simulink model "Modelo_con_no_linealidades_filtro_sensor"  (R2020a)
settings: Solver=ode15s  StartTime=0.0  StopTime=10  FixedStep=0.001  MaxStep=0.0001  RelTol=1e-3
undefined symbols (not defined in the file): A, Amp, B, ba, Cc, D, den_anti, den_des, den_mems, den_piezo, f0, fs, g, I_max, K_motor_virtual, ksi, ksia, L, num_anti, num_des, num_mems, num_piezo, R, R_control, sens_mems, sens_piezo, v0, Vcc, x0, ZOH
libraries: simulink x2, dsparch4 x2, simulink_extras x2, dspstat3 x1
settings Model: Creator=Noxi-PC  LastModifiedBy=Noxi-PC

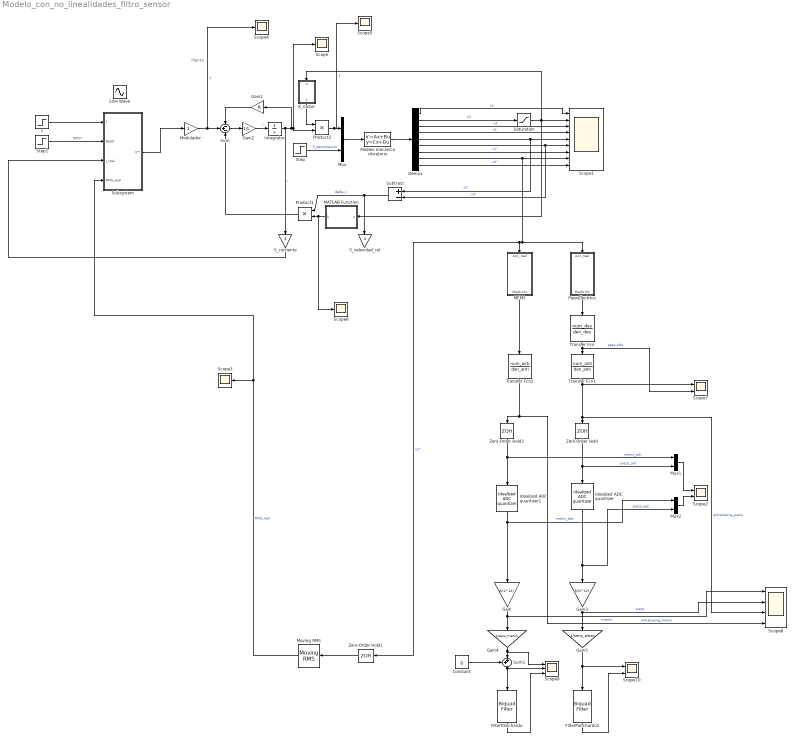
== system Modelo_con_no_linealidades_filtro_sensor ==
  note: Planta
  " PiezoElectrico" : Subsystem
  Constant : Constant  Value=g
  Demux : Demux  Outputs=9
  FilterPanchardo : dsparch4/Biquad Filter  Tag=BlockMethodSubSystem  FilterSource=Dialog parameters  CoeffSource=Specify via dialog  FilterObject=BQF  IIRFiltStruct=Direct form II  BiQuadCoeffs=[1 0 -1 1 -1.99807727905716614 0.999282800663373716;1 0 -1 1 -1.9986275895624166 0.999418888027123309;1 0 -1 1 -1.9966899219313865 0.997885027756237442;1 0 -1 1 -1.99747521879656054 0.998272398940524885;1 0 -1 1 -1.99541616433952562 0.996591907571157343;1 0 -1 1 -1.9963625045137694 0.997171843682499337;1 0 -1 1 -1.99431507711195533 0.995463604360754095;1 0 -1 1 -1.99532069965140524 0.996148326323776701;1 0 -1 1 -1.9934341214911746 0.99454907245261337;1 0 -1 1 -1.99438289828679416 0.995234669646854031;1 0 -1 1 -1.99280645736345186 0.993883243383688608;1 0 -1 1 -1.99358390398571439 0.994465232331816384;1 0 -1 1 -1.9924496211917011 0.993485563750365785;1 0 -1 1 -1.99295923065970682 0.993874854162103194;1 0 -1 1 -1.99236572677773305 0.993360052380677261;1 0 -1 1 -1.99254312887680385 0.993496835183648508]  ScaleValues=[0.00331146928203063717;0.00331146928203063717;0.00330936361502479461;0.00330936361502479461;0.00330738378960852624;0.00330738378960852624;0.00330560502842379075;0.00330560502842379075;0.00330409457240921122;0.00330409457240921122;0.00330290926614940734;0.00330290926614940734;0.00330209355456580114;0.00330209355456580114;0.00330167794092392887;0.00330167794092392887;1]  IC=0  ICnum=0  ICden=0  a0Flag=Warning  optimizeScaleValues=on  ScaleValueMode=Specify via input port (g)  InputProcessing=Columns as channels (frame based)  roundingMode=Floor  overflowMode=off  scaleValueFracLength=14  denProdOutputFracLength=30  denAccumFracLength=30  secondMemoryFracLength=15
  FilterPanchardo1 : dsparch4/Biquad Filter  Tag=BlockMethodSubSystem  FilterSource=Dialog parameters  CoeffSource=Specify via dialog  FilterObject=BQF  IIRFiltStruct=Direct form II  BiQuadCoeffs=[1 0 -1 1 -1.99807727905716614 0.999282800663373716;1 0 -1 1 -1.9986275895624166 0.999418888027123309;1 0 -1 1 -1.9966899219313865 0.997885027756237442;1 0 -1 1 -1.99747521879656054 0.998272398940524885;1 0 -1 1 -1.99541616433952562 0.996591907571157343;1 0 -1 1 -1.9963625045137694 0.997171843682499337;1 0 -1 1 -1.99431507711195533 0.995463604360754095;1 0 -1 1 -1.99532069965140524 0.996148326323776701;1 0 -1 1 -1.9934341214911746 0.99454907245261337;1 0 -1 1 -1.99438289828679416 0.995234669646854031;1 0 -1 1 -1.99280645736345186 0.993883243383688608;1 0 -1 1 -1.99358390398571439 0.994465232331816384;1 0 -1 1 -1.9924496211917011 0.993485563750365785;1 0 -1 1 -1.99295923065970682 0.993874854162103194;1 0 -1 1 -1.99236572677773305 0.993360052380677261;1 0 -1 1 -1.99254312887680385 0.993496835183648508]  ScaleValues=[0.00331146928203063717;0.00331146928203063717;0.00330936361502479461;0.00330936361502479461;0.00330738378960852624;0.00330738378960852624;0.00330560502842379075;0.00330560502842379075;0.00330409457240921122;0.00330409457240921122;0.00330290926614940734;0.00330290926614940734;0.00330209355456580114;0.00330209355456580114;0.00330167794092392887;0.00330167794092392887;1]  IC=0  ICnum=0  ICden=0  a0Flag=Warning  optimizeScaleValues=on  ScaleValueMode=Specify via input port (g)  InputProcessing=Columns as channels (frame based)  roundingMode=Floor  overflowMode=off  scaleValueFracLength=14  denProdOutputFracLength=30  denAccumFracLength=30  secondMemoryFracLength=15
  Gain : Gain  Gain=5/(2^12)
  Gain1 : Gain  Gain=R
  Gain2 : Gain  Gain=1/L
  Gain3 : Gain  Gain=5/(2^12)
  Gain4 : Gain  Gain=1/sens_mems
  Gain5 : Gain  Gain=1/sens_piezo
  Idealized ADC quantizer : simulink_extras/Additional Discrete/Idealized ADC quantizer  NumberOfConverterBits=12  Vmin=-2.5  Vmax=2.5  OutputDataType=int16  OutputNegativeValues=on
  Idealized ADC quantizer1 : simulink_extras/Additional Discrete/Idealized ADC quantizer  NumberOfConverterBits=12  Vmin=0  Vmax=3.3  OutputDataType=int16  OutputNegativeValues=on
  Integrator : Integrator
  K_motor : MATLAB Function  TreatAsAtomicUnit=on
  MATLAB Function : MATLAB Function  TreatAsAtomicUnit=on
  MEMS : Subsystem
  Modelo mecánico vibratorio : StateSpace  A=A  B=B  C=Cc  D=D  InitialCondition=[x0,v0]
  Modulador : Gain
  Moving RMS : dspstat3/Moving RMS  Method=Sliding window  ForgettingFactorPort=off  SpecifyWindowLength=on  WindowLength=Ventana  ForgettingFactor=0.99  SimulateUsing=Code generation
      settings: SourceProductBaseCode=DS
  Mux : Mux  Inputs=2
  Mux1 : Mux  Inputs=2
  Mux2 : Mux  Inputs=2
  Product1 : Product
  Product2 : Product
  S_corriente : Gain
  S_velocidad_rel : Gain
  Saturation : Saturate  UpperLimit=12.7e-3  LowerLimit=-12.7e-3
  Scope{,3..6} (5 alike) : Scope
  Scope1 : Scope  NumInputPorts=9
  Scope10 : Scope  NumInputPorts=2
  Scope2 : Scope  NumInputPorts=2
  Scope7 : Scope  NumInputPorts=2
  Scope8 : Scope  NumInputPorts=4
  Scope9 : Scope  NumInputPorts=3
  Sine Wave : Sin  Amplitude=5  Frequency=2*pi*f0  SampleTime=0
  Step : Step  Time=3  After=0  SampleTime=0
  Step1 : Step  After=Amp/sqrt(2)  SampleTime=0
  Subsystem : Subsystem
  Subtract : Sum  Inputs=+-
  Sum : Sum  Inputs=-+-
  Sum1 : Sum  Inputs=++|
  Transfer Fcn : TransferFcn  Numerator=num_des  Denominator=den_des
  Transfer Fcn1 : TransferFcn  Numerator=num_anti  Denominator=den_anti
  Transfer Fcn2 : TransferFcn  Numerator=num_anti  Denominator=den_anti
  Zero-Order Hold : ZeroOrderHold  SampleTime=1/fs
  Zero-Order Hold1 : ZeroOrderHold  SampleTime=ZOH
  Zero-Order Hold2 : ZeroOrderHold  SampleTime=1/fs
  f : Step  Time=0  After=f0  SampleTime=0
  wires:
  Modelo mecánico vibratorio/1 -> Demux/1
  Demux/1 -> Scope1/1  "x1"
  Demux/2 -> Saturation/1  "x2"
  Demux/3 -> Scope1/3  "x3"
  Demux/4 -> Scope1/4  "x1'"
  Demux/5 -> Scope1/5, Subtract/1  "x2'"
  Demux/6 -> Scope1/6, Subtract/2  "x3'"
  Demux/7 -> Scope1/7  "x1''"
  Demux/8 -> " PiezoElectrico"/1(Acc_real), Zero-Order Hold1/1, MEMS/1(Acc_real), Scope1/8  "x2''"
  Demux/9 -> Scope1/9  "x3''"
  Mux/1 -> Modelo mecánico vibratorio/1
  Sum/1 -> Gain2/1
  Integrator/1 -> S_corriente/1, Product2/2, Scope/1, Gain1/1  "i"
  Gain1/1 -> Sum/1
  Gain2/1 -> Integrator/1  "i'"
  Step/1 -> Mux/2  "F_perturbación"
  Product1/1 -> Sum/3
  Subtract/1 -> Product1/1, S_velocidad_rel/1  "delta_v"
  Modulador/1 -> Scope4/1, Sum/2  "V"
  Moving RMS/1 -> Subsystem/4(RMS_real), Scope3/1  "RMS_real"
  Saturation/1 -> K_motor/1(u), MATLAB Function/1(u), Scope1/2
  Product2/1 -> Scope5/1, Mux/1  "F"
  K_motor/1(k) -> Product2/1
  MATLAB Function/1(k) -> Scope6/1, Product1/2
  f/1 -> Subsystem/1(f)
  Step1/1 -> Subsystem/2(RMS*)  "RMS*"
  S_corriente/1 -> Subsystem/3(i_real)
  Subsystem/1(V*') -> Modulador/1
  " PiezoElectrico"/1(Medición) -> Transfer Fcn/1
  Transfer Fcn/1 -> Scope7/2, Transfer Fcn1/1  "pasa-alto"
  Transfer Fcn1/1 -> Scope8/3, Zero-Order Hold/1, Scope7/1  "antialiasing_piezo"
  Zero-Order Hold/1 -> Mux1/2, Idealized ADC quantizer/1  "piezo_zoh"
  MEMS/1(Medición) -> Transfer Fcn2/1
  Transfer Fcn2/1 -> Scope8/4, Zero-Order Hold2/1  "antialiasing_mems"
  Zero-Order Hold2/1 -> Mux1/1, Idealized ADC quantizer1/1  "mems_zoh"
  Mux1/1 -> Scope2/1
  Idealized ADC quantizer/1 -> Mux2/2, Gain3/1  "piezo_adc"
  Idealized ADC quantizer1/1 -> Gain/1, Mux2/1  "mems_adc"
  Mux2/1 -> Scope2/2
  Gain/1 -> Scope8/1, Gain4/1  "mems"
  Gain3/1 -> Scope8/2, Gain5/1  "piezo"
  Sum1/1 -> Scope9/2, FilterPanchardo/1
  Gain4/1 -> Scope9/1, Sum1/2
  Constant/1 -> Sum1/1
  Gain5/1 -> FilterPanchardo1/1, Scope10/1
  FilterPanchardo1/1 -> Scope10/2
  FilterPanchardo/1 -> Scope9/3
  Zero-Order Hold1/1 -> Moving RMS/1

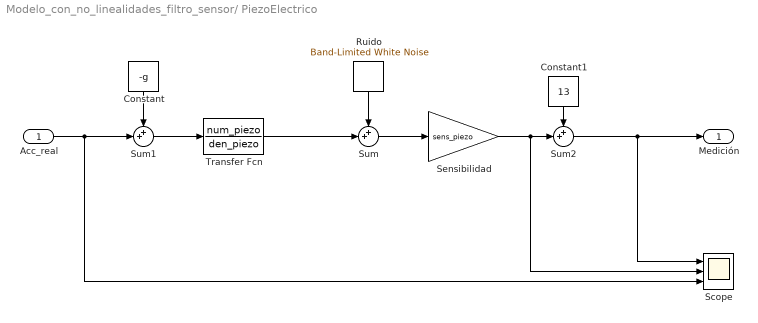
== system Modelo_con_no_linealidades_filtro_sensor/ PiezoElectrico ==
  Acc_real : Inport
  Constant : Constant  Value=-g
  Constant1 : Constant  Value=13
  Ruido : simulink/Sources/Band-Limited White Noise  Cov=NoisePower_piezo  Ts=1/fs  seed=[23341]
  Scope : Scope  NumInputPorts=3
  Sensibilidad : Gain  Gain=sens_piezo
  Sum : Sum  Inputs=++|
  Sum1 : Sum  Inputs=++|
  Sum2 : Sum  Inputs=++|
  Transfer Fcn : TransferFcn  Numerator=num_piezo  Denominator=den_piezo
  Medición : Outport
  wires:
  Transfer Fcn/1 -> Sum/2
  Ruido/1 -> Sum/1
  Constant/1 -> Sum1/1
  Sum1/1 -> Transfer Fcn/1
  Acc_real/1 -> Scope/3, Sum1/2
  Sum/1 -> Sensibilidad/1
  Constant1/1 -> Sum2/1
  Sensibilidad/1 -> Scope/2, Sum2/2
  Sum2/1 -> Medición/1, Scope/1

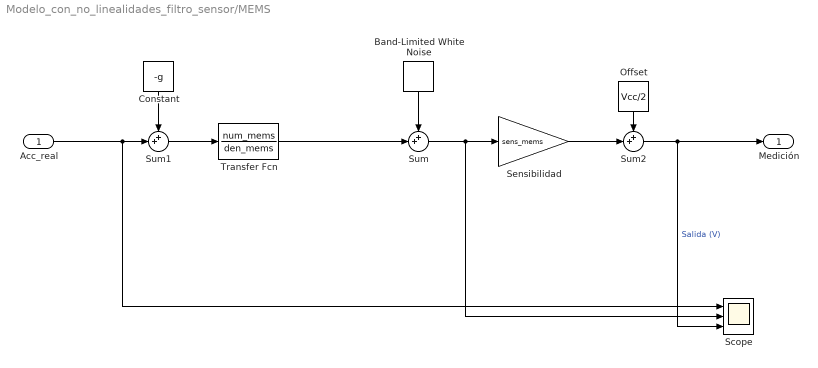
== system Modelo_con_no_linealidades_filtro_sensor/MEMS ==
  Acc_real : Inport
  Band-Limited White Noise : simulink/Sources/Band-Limited White Noise  Cov=NoisePower_mems  Ts=1/fs  seed=[23341]
  Constant : Constant  Value=-g
  Offset : Constant  Value=Vcc/2
  Scope : Scope  NumInputPorts=3
  Sensibilidad : Gain  Gain=sens_mems
  Sum : Sum  Inputs=++|
  Sum1 : Sum  Inputs=++|
  Sum2 : Sum  Inputs=++|
  Transfer Fcn : TransferFcn  Numerator=num_mems  Denominator=den_mems
  Medición : Outport
  wires:
  Sum1/1 -> Transfer Fcn/1
  Constant/1 -> Sum1/1
  Acc_real/1 -> Scope/1, Sum1/2
  Band-Limited White Noise/1 -> Sum/1
  Transfer Fcn/1 -> Sum/2
  Sum/1 -> Scope/2, Sensibilidad/1
  Sensibilidad/1 -> Sum2/2
  Offset/1 -> Sum2/1
  Sum2/1 -> Scope/3, Medición/1  "Salida (V)"

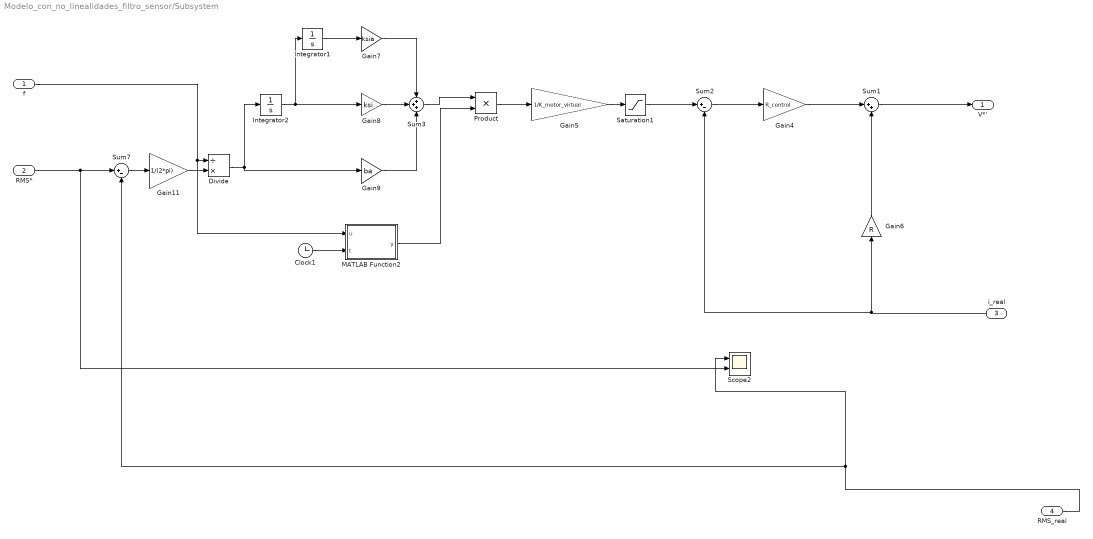
== system Modelo_con_no_linealidades_filtro_sensor/Subsystem ==
  f : Inport
  RMS* : Inport  Port=2
  i_real : Inport  Port=3
  RMS_real : Inport  Port=4
  Clock1 : Clock
  Divide : Product  Inputs=/*
  Gain11 : Gain  Gain=1/(2*pi)
  Gain4 : Gain  Gain=R_control
  Gain5 : Gain  Gain=1/K_motor_virtual
  Gain6 : Gain  Gain=R
  Gain7 : Gain  Gain=ksia
  Gain8 : Gain  Gain=ksi
  Gain9 : Gain  Gain=ba
  Integrator1 : Integrator
  Integrator2 : Integrator
  MATLAB Function2 : MATLAB Function  TreatAsAtomicUnit=on
  Product : Product
  Saturation1 : Saturate  UpperLimit=I_max  LowerLimit=-I_max
  Scope2 : Scope  NumInputPorts=2
  Sum1 : Sum  Inputs=|++
  Sum2 : Sum  Inputs=|+-
  Sum3 : Sum  Inputs=+++
  Sum7 : Sum  Inputs=|+-
  V*' : Outport
  wires:
  Integrator1/1 -> Gain7/1
  Integrator2/1 -> Integrator1/1, Gain8/1
  RMS_real/1 -> Scope2/1, Sum7/2
  RMS*/1 -> Scope2/2, Sum7/1
  Gain8/1 -> Sum3/2
  Gain5/1 -> Saturation1/1
  Gain4/1 -> Sum1/1
  Sum2/1 -> Gain4/1
  Gain9/1 -> Sum3/3
  Sum7/1 -> Gain11/1
  i_real/1 -> Gain6/1, Sum2/2
  f/1 -> MATLAB Function2/1(u), Divide/1
  Gain6/1 -> Sum1/2
  Sum3/1 -> Product/1
  Product/1 -> Gain5/1
  Saturation1/1 -> Sum2/1
  Gain11/1 -> Divide/2
  Gain7/1 -> Sum3/1
  Divide/1 -> Gain9/1, Integrator2/1
  Clock1/1 -> MATLAB Function2/2(t)
  MATLAB Function2/1(y) -> Product/2
  Sum1/1 -> V*'/1

== matlab function Modelo_con_no_linealidades_filtro_sensor/MATLAB Function ==
  data: u input; k output
function k= fcn(u)
coefs = [1883883250149.81,121220914.941173,-604988778.285297,-369001.905871325,-43371.4523559472,-47.4444922489166,51.4222931299995];

k = coefs(1)*u^6+coefs(2)*u^5+coefs(3)*u^4+coefs(4)*u^3+coefs(5)*u^2+coefs(6)*u^1+coefs(7);

== matlab function Modelo_con_no_linealidades_filtro_sensor/Subsystem/MATLAB Function2 ==
  data: u input; y output; t input
function y = fcn(u,t)

y = sin(2*pi*u*t);

== matlab function Modelo_con_no_linealidades_filtro_sensor/K_motor ==
  data: u input; k output
function k = fcn(u)
coefs = [1.88388325014986e-06,1.21220914940963e-07,-0.000604988778285308,-0.000369001905871298,-0.0433714523559467,-0.0474444922489168,51.4222931299995];

k = coefs(1)*u^6+coefs(2)*u^5+coefs(3)*u^4+coefs(4)*u^3+coefs(5)*u^2+coefs(6)*u^1+coefs(7);
